simulink model "phasebetter"  (R2020a)
settings: Solver=VariableStepAuto  StartTime=0.0  StopTime=0.0001  RelTol=1e-3
libraries: simulink x3, dsparch4 x3, dspadpt3 x3
settings Model: Creator=verty  LastModifiedBy=verty

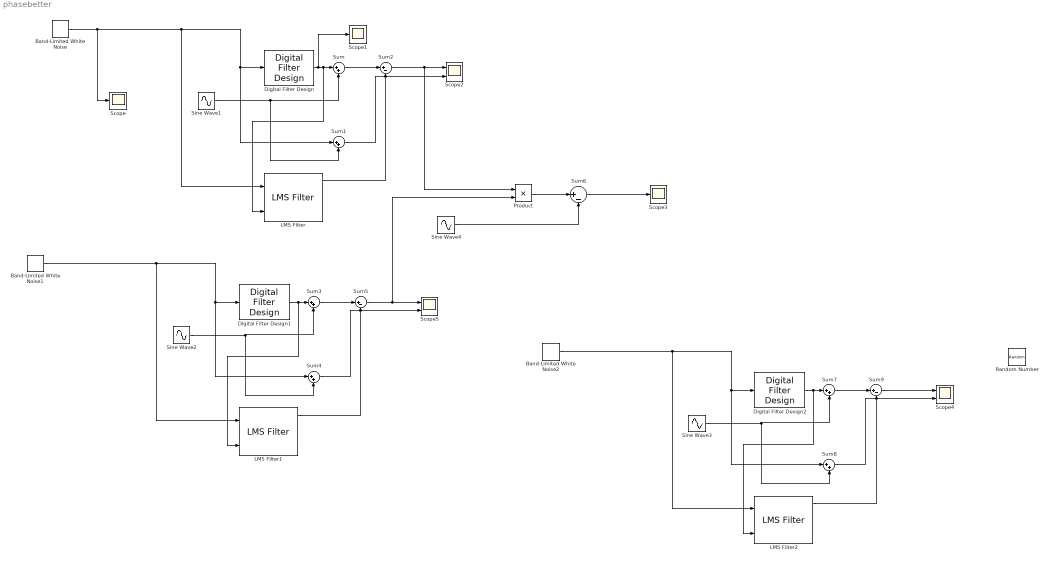
== system phasebetter ==
  Band-Limited White Noise : simulink/Sources/Band-Limited White Noise  Cov=[0.0000000001]  Ts=0.0000000001  seed=[23341]
  Band-Limited White Noise1 : simulink/Sources/Band-Limited White Noise  Cov=[0.0000000001]  Ts=0.0000000001  seed=[23341]
  Band-Limited White Noise2 : simulink/Sources/Band-Limited White Noise  Cov=[0.0000000001]  Ts=0.0000000001  seed=[23341]
  Digital Filter Design : dsparch4/Digital Filter Design  mwdsp_browser_bugfix_var=off
  Digital Filter Design1 : dsparch4/Digital Filter Design  mwdsp_browser_bugfix_var=off
  Digital Filter Design2 : dsparch4/Digital Filter Design  mwdsp_browser_bugfix_var=off
  LMS Filter : dspadpt3/LMS Filter  Algo=Normalized LMS  L=1000  stepflag=Dialog  mu=0.1  leakage=1.0  ic=0  Adapt=off  resetflag=None  weights=on  addnparflag=off  roundingMode=Floor  overflowMode=off
      settings: SourceProductBaseCode=DS
  LMS Filter1 : dspadpt3/LMS Filter  Algo=Normalized LMS  L=1000  stepflag=Dialog  mu=0.1  leakage=1.0  ic=0  Adapt=off  resetflag=None  weights=on  addnparflag=off  roundingMode=Floor  overflowMode=off
      settings: SourceProductBaseCode=DS
  LMS Filter2 : dspadpt3/LMS Filter  Algo=Normalized LMS  L=1000  stepflag=Dialog  mu=0.1  leakage=1.0  ic=0  Adapt=off  resetflag=None  weights=on  addnparflag=off  roundingMode=Floor  overflowMode=off
      settings: SourceProductBaseCode=DS
  Product : Product
  Random Number : RandomNumber  SampleTime=0.1
  Scope : Scope
  Scope1 : Scope
  Scope2 : Scope  NumInputPorts=2
  Scope3 : Scope
  Scope4 : Scope  NumInputPorts=2
  Scope5 : Scope  NumInputPorts=2
  Sine Wave1 : Sin  Amplitude=10  Frequency=48000000  Phase=1.57079633  SampleTime=0.0000000001  VectorParams1D=off
  Sine Wave2 : Sin  Amplitude=10  Frequency=50000000  Phase=0.67  SampleTime=0.0000000001  VectorParams1D=off
  Sine Wave3 : Sin  Amplitude=10  Frequency=50000000  Phase=0.67  SampleTime=0.0000000001  VectorParams1D=off
  Sine Wave4 : Sin  Amplitude=50  Frequency=98000000  Phase=0.67  SampleTime=0.0000000001  VectorParams1D=off
  Sum{,1,3..4,7..8} (6 alike) : Sum  Inputs=|++
  Sum{2,5..6,9} (4 alike) : Sum  Inputs=|+-
  wires:
  Sine Wave1/1 -> Sum/2, Sum1/2
  Digital Filter Design/1 -> Scope1/1, LMS Filter/2, Sum/1
  Sum1/1 -> Scope2/2
  Band-Limited White Noise/1 -> Scope/1, LMS Filter/1, Digital Filter Design/1, Sum1/1
  Sum/1 -> Sum2/1
  LMS Filter/1 -> Sum2/2
  LMS Filter1/1 -> Sum5/2
  Sum5/1 -> Product/2, Scope5/1
  Sum3/1 -> Sum5/1
  Sum4/1 -> Scope5/2
  Band-Limited White Noise1/1 -> LMS Filter1/1, Digital Filter Design1/1, Sum4/1
  Digital Filter Design1/1 -> LMS Filter1/2, Sum3/1
  Sine Wave2/1 -> Sum3/2, Sum4/2
  Sum2/1 -> Product/1, Scope2/1
  Product/1 -> Sum6/1
  Sum6/1 -> Scope3/1
  Sine Wave4/1 -> Sum6/2
  LMS Filter2/1 -> Sum9/2
  Digital Filter Design2/1 -> LMS Filter2/2, Sum7/1
  Sum9/1 -> Scope4/1
  Sum8/1 -> Scope4/2
  Sum7/1 -> Sum9/1
  Sine Wave3/1 -> Sum7/2, Sum8/2
  Band-Limited White Noise2/1 -> LMS Filter2/1, Digital Filter Design2/1, Sum8/1
